simulink model "flyback_dt"  (R2021b)
settings: Solver=FixedStepAuto  StartTime=0.0  StopTime=100e-06  FixedStep=1e-07  RelTol=1e-3
model workspace (MAT data in the model file):
  SDO_OutputTimes = [0; 0.0062; 0.0124; 0.0186; 0.0248; 0.031; 0.0372; 0.0434; 0.0496; 0.0558; 0.062; 0.0682; 0.0744; 0.0806; 0.0868; 0.093; 0.0992; 0.1054; 0.1116; 0.1178; 0.124; 0.1302; 0.1364; 0.1426; 0.1488; 0.155; 0.1612; 0.1674; 0.1736; 0.1798; 0.186; 0.1922; 0.1984; 0.2046; 0.2108; 0.217; 0.2232; 0.2294; 0.2356; 0.2418; 0.248; 0.2542; 0.2604; 0.2666; 0.2728; 0.279; 0.2852; 0.2914; 0.2976; 0.3038; 0.31; 0.3162; 0.3224; 0.3286; 0.3348; 0.341; 0.3472; 0.3534; 0.3596; 0.3658; 0.372; 0.3782; 0.3844; 0.3906; 0.3968; 0.403; 0.4092]
values from neighbouring files (symbols this model uses):
  L = 36.5e-6    (= 3.65e-05)    [datasetCreation.m]
  M = 1.5735e-5    (= 1.5735e-05)    [datasetCreation.m]
  R = resultTable.R(i)    [datasetCreation.m]
libraries: fl_lib x16, nesl_utility x4, ee_lib x3
settings Model: Creator=JustusPC  LastModifiedBy=Marco Milanesi
settings DataIOCC: ExternalInput=tp4744a1d6_6ac0_4d04_809d_c98f3a307d58(1)  OutputOption=AdditionalOutputTimes  OutputTimes=SDO_OutputTimes  ReturnWorkspaceOutputsName=SDOSimTest_Log
settings DebuggingCC: UnconnectedInputMsg=none  UnconnectedOutputMsg=none  UnconnectedLineMsg=none
settings ModelReferenceCC: EnableRefExpFcnMdlSchedulingChecks=off
settings RTWCC: DLArmComputeVersion=20.02.1

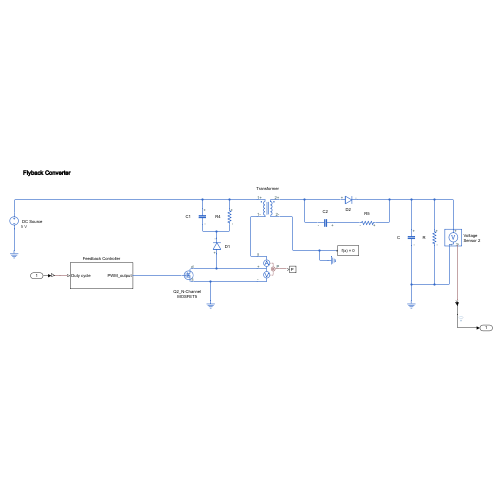
[thumbnail: Simulink's stored preview of the top-level diagram]
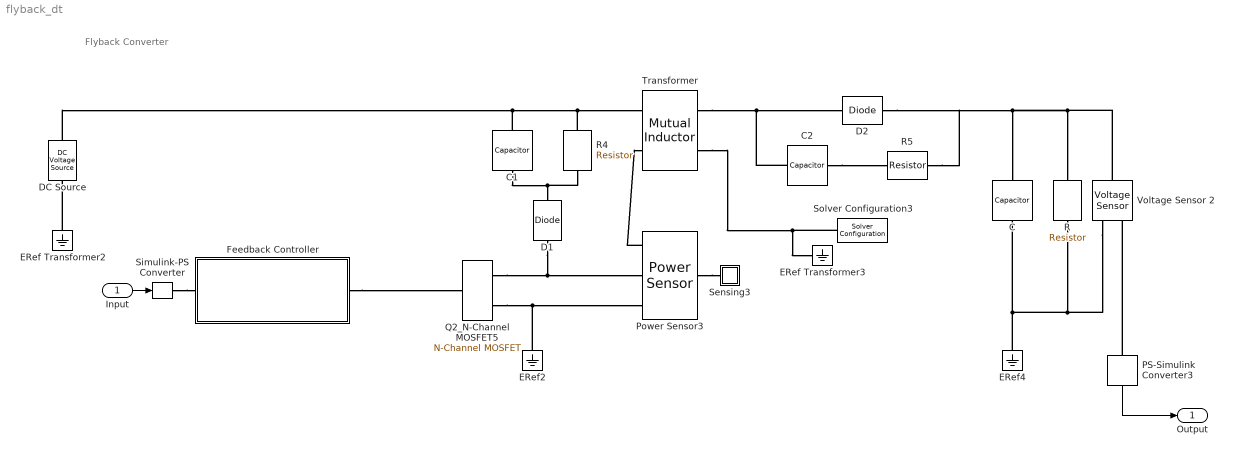
== system flyback_dt ==
  note: Flyback Converter
  Input : Inport
  C : fl_lib/Electrical/Electrical Elements/Capacitor  c=C F  r=1e-6 Ohm  g=0 1/Ohm  i_specify=off  i_priority=None  i=0 A  i_nominal_specify=off  i_nominal_unit=A  i_nominal_value=1  v_specify=off  v_priority=None  v=0 V  v_nominal_specify=off  v_nominal_unit=V  v_nominal_value=1  vc_specify=off  vc_priority=High  vc=0 V  vc_nominal_specify=off  vc_nominal_unit=V  vc_nominal_value=1
  C1 : fl_lib/Electrical/Electrical Elements/Capacitor  c=100 pF  r=1e-6 Ohm  g=0 1/Ohm  i_specify=off  i_priority=None  i=0 A  i_nominal_specify=off  i_nominal_unit=A  i_nominal_value=1  v_specify=off  v_priority=None  v=0 V  v_nominal_specify=off  v_nominal_unit=V  v_nominal_value=1  vc_specify=off  vc_priority=High  vc=0 V  vc_nominal_specify=off  vc_nominal_unit=V  vc_nominal_value=1
  C2 : fl_lib/Electrical/Electrical Elements/Capacitor  c=1 nF  r=1e-6 Ohm  g=0 1/Ohm  i_specify=off  i_priority=None  i=0 A  i_nominal_specify=off  i_nominal_unit=A  i_nominal_value=1  v_specify=off  v_priority=None  v=0 V  v_nominal_specify=off  v_nominal_unit=V  v_nominal_value=1  vc_specify=off  vc_priority=High  vc=0 V  vc_nominal_specify=off  vc_nominal_unit=V  vc_nominal_value=1
  D1 : fl_lib/Electrical/Electrical Elements/Diode  Vf=0.25 V  Ron=1 Ohm  Goff=1e-08 1/Ohm  i_specify=off  i_priority=High  i=0 A  i_nominal_specify=off  i_nominal_unit=A  i_nominal_value=1  v_specify=off  v_priority=High  v=0 V  v_nominal_specify=off  v_nominal_unit=V  v_nominal_value=1
  D2 : fl_lib/Electrical/Electrical Elements/Diode  Vf=0.25 V  Ron=1 Ohm  Goff=1e-08 1/Ohm  i_specify=off  i_priority=High  i=0 A  i_nominal_specify=off  i_nominal_unit=A  i_nominal_value=1  v_specify=off  v_priority=High  v=0 V  v_nominal_specify=off  v_nominal_unit=V  v_nominal_value=1
  DC Source : fl_lib/Electrical/Electrical Sources/DC Voltage Source  v0=5 V
      settings: AttributesFormatString=%<v0> %<v0_unit>
  ERef Transformer2 : fl_lib/Electrical/Electrical Elements/Electrical Reference
  ERef Transformer3 : fl_lib/Electrical/Electrical Elements/Electrical Reference
  ERef2 : fl_lib/Electrical/Electrical Elements/Electrical Reference
  ERef4 : fl_lib/Electrical/Electrical Elements/Electrical Reference
  Feedback Controller : Subsystem
  PS-Simulink Converter3 : nesl_utility/PS-Simulink Converter  PhysicalDomain=network_engine_domain  SubClassName=ps_output  LeftPortType=input  RightPortType=output  PseudoPeriodic=off  Frequencies=[]  Unit=1  AffineConversion=off
      settings: SourceProductBaseCode=PW,SS
  Power Sensor3 : ee_lib/Sensors & Transducers/Power Sensor  measurement_type=2  averaging_period=1/10e5 s
      settings: SourceProductBaseCode=PS
  Q2_N-Channel MOSFET5 : ee_lib/Semiconductors & Converters/N-Channel MOSFET  paramTerminal=ee.enum.mosfet.numberOfTerminals.three  parameterization=ee.enum.mosfet.parameterization.datasheet  Beta=5 A/V^2  Rds=0.01 Ohm  Id=100 A  Vgs=5 V  Vth=2 V  Vth0=1.7 V  lam=0 1/V  gamma_vth=0.5 V^(1/2)  phib=0.5 V  Vth1=1.9071 V  Vbs1=-1 V  Vth2=2.066 V  Vbs2=-2 V  Tmeas=25 degC  Vgs_vec=[-.5, 2, 3, 4, 5] V  Vds_vec=[0, 2, 4, 8, 12, 16, 20] V  Vbs_vec=[0, -4, -6, -12] V  T_vec=[25, 125] degC  Vth_vec=[.4, 1.2, 1.4, 1.45] V  Vth_mat=[.4, .35; 1.2, 1.15; 1.4, 1.35; 1.45, 1.4] V  Ids_mat=[0, 0, 0, 0, 0, 0, 0; 0, .003, .0038, .0043, .0046, .0048, .0049; 0, .0055, .008, .009, .0095, .01, .0101; 0, .0115, .016, .018, .019, .0195, .02; 0, .0152, .0225, .0265, .028, .0295, .03] A  Ids_mat0=[0, 0, 0, 0, 0, 0, 0; 0, .003, .0038, .0043, .0046, .0048, .0049; 0, .0055, .008, .009, .0095, .01, .0101; 0, .0115, .016, .018, .019, .0195, .02; 0, .0152, .0225, .0265, .028, .0295, .03] A  Ids_mat_3D=zeros(5, 7, 2) A  Ids_mat_3D0=zeros(5, 7, 2) A  IV_table_symmetry=ee.enum.mosfet.symmetricNIV.no  RS=0.001 Ohm  RD=0.001 Ohm  RB=0.001 Ohm  C_param=ee.enum.mosfet.capacitanceParam.fixedciss  C_GS=270 pF  C_GD=80 pF  C_DS=0 pF  C_iss=700 pF  C_rss=160 pF  C_oss=0 pF  charge_linearity_param=ee.enum.mosfet.cgdLinearity.constant  C_OX=200 pF  V_C_OX=-0.5 V  charge_linearity_param_vgb=ee.enum.mosfet.cgbLinearity.instantly  C_iss_vec=[ 720 700 590 470 390 310 ] pF  C_rss_vec=[ 450 400 300 190 95 55 ] pF  C_oss_vec=[ 900 810 690 420 270 170 ] pF  C_GS_vec=[ 270 300 290 280 295 255 ] pF  C_GD_vec=[ 450 400 300 190 95 55 ] pF  C_DS_vec=[ 450 410 390 230 175 115 ] pF  C_Vds_vec=[ 0.1 0.3 1 3 10 30 ] V  V_GS_for_cap_data=NaN V  Di_param=ee.enum.mosfet.diodeParam.exponential  IsDiode=0 A  Vbi=0.6 V  n=1  Cj0Diode=0 pF  TT=50e-9 s  Tmeas_dio=25 degC  TableTypeNoT=ee.enum.mosfet.tableType.IfMat  TableType=ee.enum.diode.tableType.IfMat  IfVec=[.07, .12, .19, 1.75, 4.24, 7.32, 11.2] A  IfMat=[.07, .12, .19, 1.75, 4.24, 7.32, 11.2; .16, .3, .72, 2.14, 4.02, 6.35, 9.12] A  VfVecV=[.9, 1.15, 1.25, 1.5, 1.75, 2.17, 2.6, 2.85] V  VfMatV=[.9, 1.15, 1.25, 1.5, 1.75, 2.17, 2.6, 2.85; .58, .68, .75, 1.1, 1.38, 1.77, 2.27, 2.7] V  TjVec=[25, 125] degC  VfVec=[.5, .7, .9, 1.3, 1.7, 2.1, 2.5] V  IfVecV=[.1, .2, .5, 1, 2, 4, 7, 10] A  prmDatasheet=ee.enum.temperatureParameterization.none  prmEquCoeff=ee.enum.temperatureParameterization.none  dVth_dT=-6 mV/K  dVth0_dT=-6 mV/K  Rds_T2=0.037 Ohm  BEXDatasheet=-1.5  BEXEquCoeff=-1.5  etaisDatasheet=3  etaisEquCoeff=3  Tmeas2=125 degC  etaisTabulated=3  TdeviceDatasheet=25 degC  TdeviceEquCoeff=25 degC  TdeviceTabulated=25 degC  thermal_network_parameterization=ee.enum.thermalNetworkTopology.junctionCase  Rth=[0, 10] K/W  Rth_Cauer=[1, 3, 10] K/W  Rth_Foster=[4, 6] K/W  thermal_mass_parameterization=ee.enum.thermalNetwork.timeconstant  thermal_mass=[0, 1] J/K  thermal_mass_Cauer=[.1, .3, 1] J/K  thermal_mass_Foster=[1.5, 3] J/K  thermal_time_constant=[0, 10] s  thermal_time_constant_Cauer=[1, 3, 10] s  thermal_time_constant_Foster=[6, 18] s  thermal_mass_initial_temperatures=[25, 25] degC  thermal_mass_initial_temperatures_Cauer=[25, 25, 25] degC  steadyState_Foster=simscape.enum.onoff.on  Tvec_initial_Foster=[25, 25, 25, 25] degC  betaref=18 A/V^2  Vfbref=-1.1 V  gamma=3.5 V^(1/2)  phib2ref=1 V  thesatref=0.4 1/V  alpha=0  Vp=5e-2 V  thesrref=0 1/V  m=8  Tref=25 degC  Rsref=2e-3 Ohm  Rdref=0.17 Ohm  Rgref=8.4 Ohm  Rbref=2e-3 Ohm  Cox=1500 pF  Cgso=100 pF  Cgdo=14 pF  Isref=5.2e-13 A  Cj0=480 pF  Tprm=1  etabet=1.3  Stvfb=5e-4 V/K  Stphib=-8.5e-4 V/K  etasat=1.04  etasr=0.65  etar=0.95  etais=3  Tsim=25 degC  T0=[25, 25] degC  T0_Cauer=[25, 25, 25] degC
  R : fl_lib/Electrical/Electrical Elements/Resistor  R=R Ohm  i_specify=off  i_priority=None  i=0 A  i_nominal_specify=off  i_nominal_unit=A  i_nominal_value=1  v_specify=off  v_priority=None  v=0 V  v_nominal_specify=off  v_nominal_unit=V  v_nominal_value=1
  R4 : fl_lib/Electrical/Electrical Elements/Resistor  R=6.8 kOhm  i_specify=off  i_priority=None  i=0 A  i_nominal_specify=off  i_nominal_unit=A  i_nominal_value=1  v_specify=off  v_priority=None  v=0 V  v_nominal_specify=off  v_nominal_unit=V  v_nominal_value=1
  R5 : fl_lib/Electrical/Electrical Elements/Resistor  R=22 Ohm  i_specify=off  i_priority=None  i=0 A  i_nominal_specify=off  i_nominal_unit=A  i_nominal_value=1  v_specify=off  v_priority=None  v=0 V  v_nominal_specify=off  v_nominal_unit=V  v_nominal_value=1
  Sensing3 : Subsystem
  Simulink-PS Converter : nesl_utility/Simulink-PS Converter  PhysicalDomain=network_engine_domain  SubClassName=ps_input  LeftPortType=input  RightPortType=output  PseudoPeriodic=off  Frequencies=[]  NoiseDistribution=none  NoiseParameters=[]  Unit=1  AffineConversion=off  FilteringAndDerivatives=provide  SimscapeFilterOrder=1  InputFilterTimeConstant=0.001  UdotUserProvided=0
      settings: SourceProductBaseCode=PW,SS
  Solver Configuration3 : nesl_utility/Solver Configuration  PhysicalDomain=network_engine_domain  SubClassName=solver  LeftPortType=input  RightPortType=generic  Tones=[]  Harmonics=[]  SimulateNoise=off  Profile=off  UseLocalSampling=off  EnableSwitchedLinearOptims=on  FrequencyDomain=off  UseCCode=off  RelTol=0.001  AbsTol=1e-06  MinStep=1e-09  ToWorkspace=off  RevertToSquareIcSolve=off  NumHomotopyIterations=100  PhasorMode=off  PhasorModeNumHarmonics=1  DoDC=off  ResidualTolerance=1e-07  UseLocalSolver=on  LocalSolverChoice=NE_BACKWARD_EULER_ADVANCER  LocalSolverSampleTime=1e-07  DoFixedCost=off  MaxNonlinIter=8  MaxModeIter=2  ComputeImpulses=off  ImpulseIterations=2  LinearAlgebra=auto  EquationFormulation=NE_TIME_EF  DelaysMemoryBudget=1024  AutomaticFiltering=on  FilteringTimeConstant=0.001  PartitionStorageMethod=AS_NEEDED  PartitionMemoryBudget=1024  PartitionMethod=FAST
      settings: SourceProductBaseCode=PW,SS
  Transformer : fl_lib/Electrical/Electrical Elements/Mutual Inductor  L1=L H  L2=L/M H  k=0.99  i1_specify=on  i1_priority=High  i1=0 A  i1_nominal_specify=off  i1_nominal_unit=A  i1_nominal_value=1  i2_specify=on  i2_priority=High  i2=0 A  i2_nominal_specify=off  i2_nominal_unit=A  i2_nominal_value=1  v1_specify=off  v1_priority=High  v1=0 V  v1_nominal_specify=off  v1_nominal_unit=V  v1_nominal_value=1  v2_specify=off  v2_priority=High  v2=0 V  v2_nominal_specify=off  v2_nominal_unit=V  v2_nominal_value=1
      settings: SourceProductBaseCode=SS  InternalSimscapePortConfiguration="{\"Bottom\":[],\"Left\":[{\"id\":\"p1\",\"label\":\"1+\",\"type\":\"foundation.electrical.electrical\"},{\"id\":\"n1\",\"label\":\"1-\",\"type\":\"foundation.electrical.electrical\"}],\"Right\":[{\"id\":\"p2\",\"label\":\"2+\",\"type\":\"foundation.electrical.electrical\"},{\"id\":\"n2\",\"label\":\"2-\",\"type\":\"foundation.electrical.electrical\"}],\"Top\":[]}"
  Voltage Sensor 2 : fl_lib/Electrical/Electrical Sensors/Voltage Sensor
  Output : Outport
  wires:
  PS-Simulink Converter3/1 -> Output/1
  Input/1 -> Simulink-PS Converter/1
  connections:
  Solver Configuration3/RConn1 -- Transformer/RConn2 -- ERef Transformer3/LConn1
  C2/RConn1 -- D2/LConn1 -- Transformer/RConn1
  Power Sensor3/RConn1 -- Sensing3/LConn1
  ERef Transformer2/LConn1 -- DC Source/RConn1
  Simulink-PS Converter/RConn1 -- Feedback Controller/LConn1
  Q2_N-Channel MOSFET5/RConn1 -- Power Sensor3/LConn2 -- D1/LConn1
  Power Sensor3/LConn1 -- Transformer/LConn2
  DC Source/LConn1 -- C1/LConn1 -- R4/LConn1 -- Transformer/LConn1
  Feedback Controller/RConn1 -- Q2_N-Channel MOSFET5/LConn1
  Q2_N-Channel MOSFET5/RConn2 -- Power Sensor3/LConn3 -- ERef2/LConn1
  Voltage Sensor 2/LConn1 -- R5/LConn1 -- D2/RConn1 -- C/LConn1 -- R/LConn1
  R/RConn1 -- Voltage Sensor 2/RConn2 -- ERef4/LConn1 -- C/RConn1
  PS-Simulink Converter3/LConn1 -- Voltage Sensor 2/RConn1
  C1/RConn1 -- R4/RConn1 -- D1/RConn1
  C2/LConn1 -- R5/RConn1

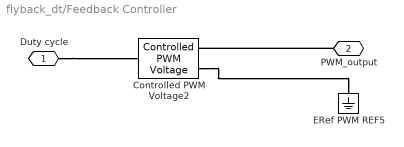
== system flyback_dt/Feedback Controller ==
  Controlled PWM Voltage2 : ee_lib/Integrated Circuits/Controlled PWM Voltage  F=50 kHz  TD=0 s  pulse_width_offset=0 s  pulse_min=0 s  pwm_or_av=1  event_type=1  sample_time=1e-6 s  Vmin=0 V  Vmax=5 V  Vm=5 V  u_min=0  u_max=1
      settings: InternalSimscapePortConfiguration="{\"Bottom\":[],\"Left\":[{\"id\":\"u\",\"label\":\"u\",\"type\":\"input\"}],\"Right\":[{\"id\":\"p2\",\"label\":\"PWM\",\"type\":\"foundation.electrical.electrical\"},{\"id\":\"n2\",\"label\":\"REF\",\"type\":\"foundation.electrical.electrical\"}],\"Top\":[]}"
  ERef PWM REF5 : fl_lib/Electrical/Electrical Elements/Electrical Reference
  Duty cycle : PMIOPort  Side=Left
  PWM_output : PMIOPort  Port=2  Side=Right
  connections:
  Controlled PWM Voltage2/RConn2 -- ERef PWM REF5/LConn1
  PWM_output/RConn1 -- Controlled PWM Voltage2/RConn1
  Duty cycle/RConn1 -- Controlled PWM Voltage2/LConn1

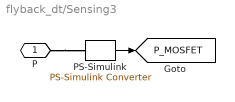
== system flyback_dt/Sensing3 ==
  PS-Simulink : nesl_utility/PS-Simulink Converter  PhysicalDomain=network_engine_domain  SubClassName=ps_output  LeftPortType=input  RightPortType=output  PseudoPeriodic=off  Frequencies=[]  Unit=W  AffineConversion=off
      settings: SourceProductBaseCode=PW,SS
  P : PMIOPort  Side=Left
  tag scope: P_MOSFET=global
  wires:
  PS-Simulink/1 -> [P_MOSFET]
  connections:
  P/RConn1 -- PS-Simulink/LConn1
